simulink library "BlockLib"  (R2014a)
settings: Solver=ode45  StartTime=0.0  StopTime=10.0  RelTol=1e-3
undefined symbols (not defined in the file or in its folder): beamSplitterReflect, beamSplitterTransmit, delay
settings Model: Creator=kunalmenda  LastModifiedBy=kunalmenda

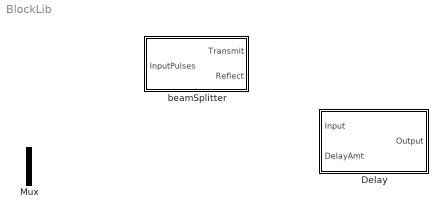
== system BlockLib ==
  Delay : Subsystem
  Mux : Mux  Inputs=2
  "beamSplitter " : Subsystem

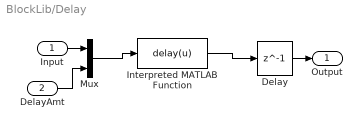
== system BlockLib/Delay ==
  Input : Inport
  DelayAmt : Inport  Port=2
  Delay : Delay  DelayLength=1  InitialCondition=0
  Interpreted MATLAB Function : MATLABFcn  MATLABFcn=delay(u)
  Mux : Mux  Inputs=2
  Output : Outport
  wires:
  Mux/1 -> Interpreted MATLAB Function/1
  Delay/1 -> Output/1
  Input/1 -> Mux/1
  Interpreted MATLAB Function/1 -> Delay/1
  DelayAmt/1 -> Mux/2

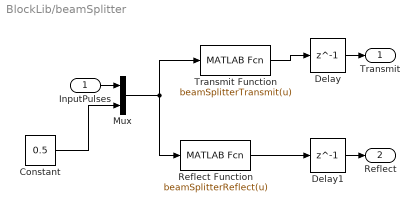
== system BlockLib/beamSplitter  ==
  InputPulses : Inport
  Constant : Constant  Value=0.5
  Delay : Delay  DelayLength=1  InitialCondition=0
  Delay1 : Delay  DelayLength=1  InitialCondition=0
  Mux : Mux  Inputs=2
  Reflect Function : MATLABFcn  MATLABFcn=beamSplitterReflect(u)
  Transmit Function : MATLABFcn  MATLABFcn=beamSplitterTransmit(u)
  Transmit : Outport
  Reflect : Outport  Port=2
  wires:
  Mux/1 -> Transmit Function/1, Reflect Function/1
  Delay1/1 -> Reflect/1
  Delay/1 -> Transmit/1
  InputPulses/1 -> Mux/1
  Constant/1 -> Mux/2
  Transmit Function/1 -> Delay/1
  Reflect Function/1 -> Delay1/1
